simulink model "topic_6"  (R2018b)
settings: Solver=FixedStepDiscrete  StartTime=0.0  StopTime=10.0  RelTol=1e-3
libraries: simulink x1
settings Model: Creator=karim  LastModifiedBy=karim
settings OptimizationCC: DefaultParameterBehavior=Inlined  EnhancedBackFolding=on  PassReuseOutputArgsAs=Individual arguments  OptimizeBlockOrder=speed  DifferentSizesBufferReuse=on  OptimizationCustomize=off
settings DebuggingCC: UnderspecifiedInitializationDetection=Classic  MergeDetectMultiDrivingBlocksExec=none  ParameterTunabilityLossMsg=error
settings ModelReferenceCC: PropagateSignalLabelsOutOfModel=off
settings SFSimCC: MATLABDynamicMemAlloc=off
settings RTWCC: SystemTargetFile=ert.tlc  GenCodeOnly=on  TemplateMakefile=ert_default_tmf  GenerateReport=on  IncludeHyperlinkInReport=on  LaunchReport=on  GenerateTraceInfo=on  GenerateTraceReport=on  GenerateTraceReportSl=on  GenerateTraceReportSf=on  GenerateTraceReportEml=on
settings CodeAppCC: ForceParamTrailComments=on  IgnoreCustomStorageClasses=off  OperatorAnnotations=on  SimulinkDataObjDesc=on  SFDataObjDesc=on  InsertBlockDesc=on
settings ERTTargetCC: TargetLangStandard=C99 (ISO)  GenerateSampleERTMain=on  SupportContinuousTime=on  InlinedParameterPlacement=NonHierarchical  ERTCustomFileTemplate=example_file_process.tlc

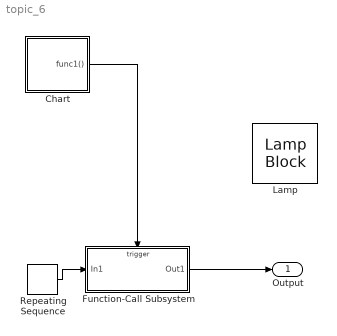
== system topic_6 ==
  Chart : Stateflow chart  TreatAsAtomicUnit=on
  Function-Call Subsystem : Subsystem  TreatAsAtomicUnit=on
  Lamp : LampBlock  WebBlockId=7  LabelPosition=Hide
  Repeating Sequence : simulink/Sources/Repeating Sequence  rep_seq_t=[0 0.5 1 1.5 2]  rep_seq_y=[0 1 1 0 0 ]
  Output : Outport
  wires:
  Chart/1(func1()) -> Function-Call Subsystem/Trigger
  Function-Call Subsystem/1(Out1) -> Output/1
  Repeating Sequence/1 -> Function-Call Subsystem/1(In1)

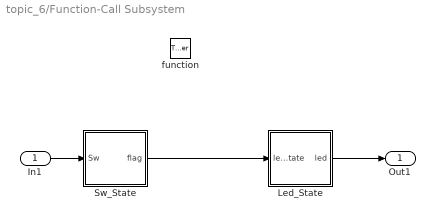
== system topic_6/Function-Call Subsystem ==
  In1 : Inport
  function : TriggerPort  TriggerType=function-call  VariantControl=Variant
  Led_State : Stateflow chart  TreatAsAtomicUnit=on
  Sw_State : Stateflow chart  TreatAsAtomicUnit=on
  Out1 : Outport
  wires:
  Sw_State/1(flag) -> Led_State/1(led_state)
  Led_State/1(led) -> Out1/1
  In1/1 -> Sw_State/1(Sw)

== stateflow chart topic_6/Function-Call Subsystem/Sw_State ==
  (default) -> (junction 7) : % Switch_State
  (junction 7) -> (junction 8) [order 1] : [Sw==1]
  (junction 7) -> (junction 9) [order 2] : {flag=0;}
  (junction 8) -> (junction 10) : {flag=1;}
  (junction 10) -> (junction 9)
  (junction 9) -> (junction 11)
  data: Sw input; flag output

== stateflow chart topic_6/Function-Call Subsystem/Led_State ==
  (default) -> (junction 9) : % Led_State
  (junction 9) -> (junction 10) [order 1] : [led_state==1]
  (junction 9) -> (junction 11) [order 2] : {led=0;}
  (junction 10) -> (junction 12) : {led=1;}
  (junction 12) -> (junction 11)
  (junction 11) -> (junction 13)
  data: data local; data1 local; led_state input; led output

== stateflow chart topic_6/Chart ==
  state CallFunction
    en:
    du:
    ex:
  (default) -> CallFunction
  CallFunction -> CallFunction : [after (5,msec)]{func1;}
  events: func1 output FUNCTION_CALL_EVENT
